simulink model "model_2020b"  (R2020b)
settings: Solver=VariableStepAuto  StartTime=0.0  StopTime=time  MaxStep=1e-3  RelTol=1e-3
values from neighbouring files (symbols this model uses):
  adj_mtx = zeros(N,N)    [main.m]
  c = 1/denominator    [main.m]
  K = B' * P / R    [main.m]
  leader_controller = place(A,B,poles)    [main.m]
  png_vector = [1 0 0 0 0 0]    [main.m]
  selected_signal = 2    [main.m]
libraries: cstblocks x8, simulink x1
settings Model: Creator=salvo  LastModifiedBy=salvo
settings DebuggingCC: UnconnectedInputMsg=none  UnconnectedOutputMsg=none  UnconnectedLineMsg=none  SFMachineParentedDataDiag=error

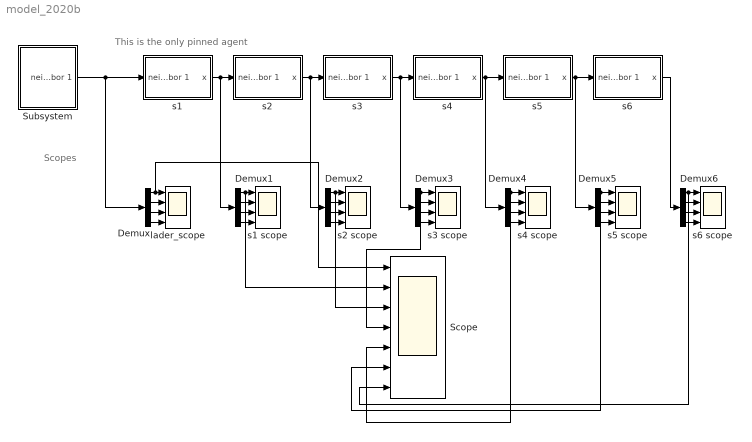
== system model_2020b ==
  note: Scopes
  note: This is the only pinned agent
  Demux{,1..6} (7 alike) : Demux
  Scope : Scope  NumInputPorts=7
  Subsystem : Subsystem
  lader_scope : Scope  NumInputPorts=4
  s1 : Subsystem
  s1 scope : Scope  NumInputPorts=4
  s2 : Subsystem
  s2 scope : Scope  NumInputPorts=4
  s3 : Subsystem
  s3 scope : Scope  NumInputPorts=4
  s4 : Subsystem
  s4 scope : Scope  NumInputPorts=4
  s5 : Subsystem
  s5 scope : Scope  NumInputPorts=4
  s6 : Subsystem
  s6 scope : Scope  NumInputPorts=4
  wires:
  Demux/1 -> Scope/1, lader_scope/1
  Demux/2 -> lader_scope/2
  Demux/3 -> lader_scope/3
  Demux/4 -> lader_scope/4
  Demux1/1 -> Scope/2, s1 scope/1
  Demux1/3 -> s1 scope/3
  Demux1/4 -> s1 scope/4
  Demux1/2 -> s1 scope/2
  s1/1(x) -> Demux1/1, s2/1(neighbor 1)
  Demux2/3 -> s2 scope/3
  Demux2/2 -> s2 scope/2
  s2/1(x) -> Demux2/1, s3/1(neighbor 1)
  Demux2/1 -> Scope/3, s2 scope/1
  Demux2/4 -> s2 scope/4
  Demux3/3 -> s3 scope/3
  Demux3/2 -> s3 scope/2
  s3/1(x) -> Demux3/1, s4/1(neighbor 1)
  Demux3/1 -> Scope/4, s3 scope/1
  Demux3/4 -> s3 scope/4
  Demux4/1 -> Scope/5, s4 scope/1
  Demux4/3 -> s4 scope/3
  s4/1(x) -> Demux4/1, s5/1(neighbor 1)
  Demux4/2 -> s4 scope/2
  Demux4/4 -> s4 scope/4
  Demux5/3 -> s5 scope/3
  s5/1(x) -> Demux5/1, s6/1(neighbor 1)
  Demux5/4 -> s5 scope/4
  Demux5/2 -> s5 scope/2
  Demux5/1 -> Scope/6, s5 scope/1
  Demux6/3 -> s6 scope/3
  Demux6/1 -> Scope/7, s6 scope/1
  s6/1(x) -> Demux6/1
  Demux6/4 -> s6 scope/4
  Demux6/2 -> s6 scope/2
  Subsystem/1(neighbor 1) -> s1/1(neighbor 1), Demux/1

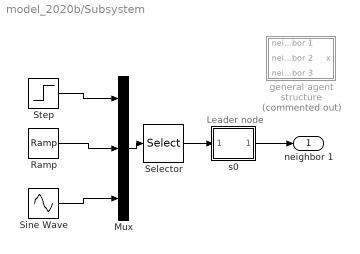
== system model_2020b/Subsystem ==
  note: Leader node
  Mux : Mux  Inputs=3
  Ramp : simulink/Sources/Ramp  slope=1  start=0  InitialOutput=0
  Selector : Selector  InputPortWidth=3  IndexOptions=Index vector (dialog)  Indices=[selected_signal]  OutputSizes=1
  Sine Wave : Sin  Amplitude=10  SampleTime=0
  Step : Step  After=2.5  SampleTime=0
  general agent structure : Subsystem  Commented=on
  s0 : Subsystem
  neighbor 1 : Outport
  wires:
  Sine Wave/1 -> Mux/3
  Selector/1 -> s0/1(In1)
  Step/1 -> Mux/1
  Mux/1 -> Selector/1
  s0/1(neighbor 1) -> neighbor 1/1
  Ramp/1 -> Mux/2

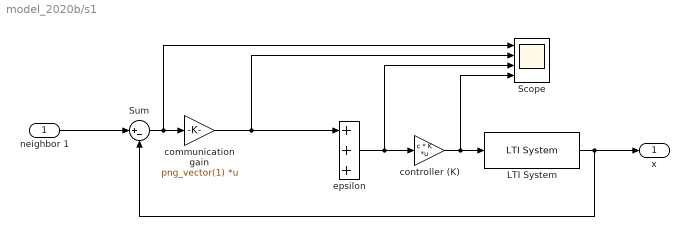
== system model_2020b/s1 ==
  neighbor 1 : Inport
  LTI System : cstblocks/LTI System  sys=sys  IC=x0_1
  Scope : Scope  NumInputPorts=4
  Sum : Sum  Inputs=|+-
  communication gain : Gain  Gain=png_vector(1)  Multiplication=Matrix(K*u)
  controller (K) : Gain  Gain=c * K  Multiplication=Matrix(K*u)
  epsilon : Sum  Inputs=+++
  x : Outport
  wires:
  LTI System/1 -> Sum/2, x/1
  controller (K)/1 -> Scope/4, LTI System/1
  neighbor 1/1 -> Sum/1
  Sum/1 -> Scope/1, communication gain/1
  epsilon/1 -> Scope/3, controller (K)/1
  communication gain/1 -> Scope/2, epsilon/1

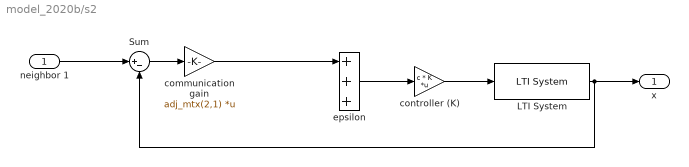
== system model_2020b/s2 ==
  neighbor 1 : Inport
  LTI System : cstblocks/LTI System  sys=sys  IC=x0_2
  Sum : Sum  Inputs=|+-
  communication gain : Gain  Gain=adj_mtx(2,1)  Multiplication=Matrix(K*u)
  controller (K) : Gain  Gain=c * K  Multiplication=Matrix(K*u)
  epsilon : Sum  Inputs=+++
  x : Outport
  wires:
  LTI System/1 -> Sum/2, x/1
  controller (K)/1 -> LTI System/1
  neighbor 1/1 -> Sum/1
  Sum/1 -> communication gain/1
  epsilon/1 -> controller (K)/1
  communication gain/1 -> epsilon/1

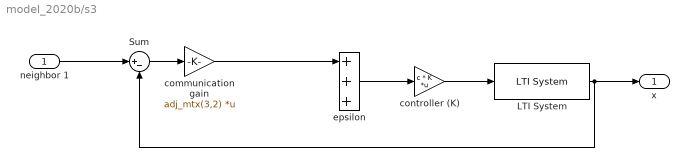
== system model_2020b/s3 ==
  neighbor 1 : Inport
  LTI System : cstblocks/LTI System  sys=sys  IC=x0_3
  Sum : Sum  Inputs=|+-
  communication gain : Gain  Gain=adj_mtx(3,2)  Multiplication=Matrix(K*u)
  controller (K) : Gain  Gain=c * K  Multiplication=Matrix(K*u)
  epsilon : Sum  Inputs=+++
  x : Outport
  wires:
  LTI System/1 -> Sum/2, x/1
  controller (K)/1 -> LTI System/1
  neighbor 1/1 -> Sum/1
  Sum/1 -> communication gain/1
  epsilon/1 -> controller (K)/1
  communication gain/1 -> epsilon/1

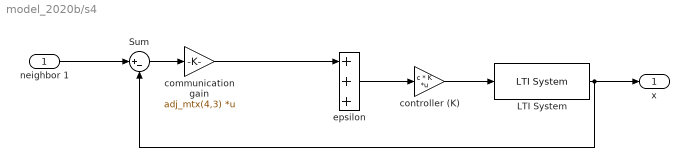
== system model_2020b/s4 ==
  neighbor 1 : Inport
  LTI System : cstblocks/LTI System  sys=sys  IC=x0_4
  Sum : Sum  Inputs=|+-
  communication gain : Gain  Gain=adj_mtx(4,3)  Multiplication=Matrix(K*u)
  controller (K) : Gain  Gain=c * K  Multiplication=Matrix(K*u)
  epsilon : Sum  Inputs=+++
  x : Outport
  wires:
  LTI System/1 -> Sum/2, x/1
  controller (K)/1 -> LTI System/1
  neighbor 1/1 -> Sum/1
  Sum/1 -> communication gain/1
  epsilon/1 -> controller (K)/1
  communication gain/1 -> epsilon/1

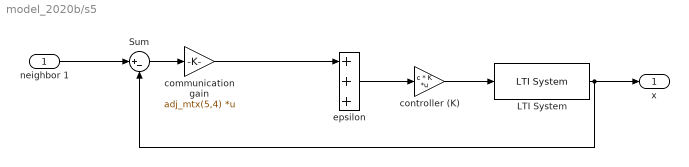
== system model_2020b/s5 ==
  neighbor 1 : Inport
  LTI System : cstblocks/LTI System  sys=sys  IC=x0_5
  Sum : Sum  Inputs=|+-
  communication gain : Gain  Gain=adj_mtx(5,4)  Multiplication=Matrix(K*u)
  controller (K) : Gain  Gain=c * K  Multiplication=Matrix(K*u)
  epsilon : Sum  Inputs=+++
  x : Outport
  wires:
  LTI System/1 -> Sum/2, x/1
  controller (K)/1 -> LTI System/1
  neighbor 1/1 -> Sum/1
  Sum/1 -> communication gain/1
  epsilon/1 -> controller (K)/1
  communication gain/1 -> epsilon/1

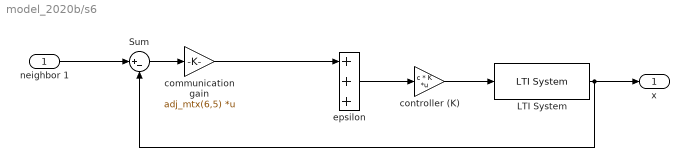
== system model_2020b/s6 ==
  neighbor 1 : Inport
  LTI System : cstblocks/LTI System  sys=sys  IC=x0_6
  Sum : Sum  Inputs=|+-
  communication gain : Gain  Gain=adj_mtx(6,5)  Multiplication=Matrix(K*u)
  controller (K) : Gain  Gain=c * K  Multiplication=Matrix(K*u)
  epsilon : Sum  Inputs=+++
  x : Outport
  wires:
  LTI System/1 -> Sum/2, x/1
  controller (K)/1 -> LTI System/1
  neighbor 1/1 -> Sum/1
  Sum/1 -> communication gain/1
  epsilon/1 -> controller (K)/1
  communication gain/1 -> epsilon/1

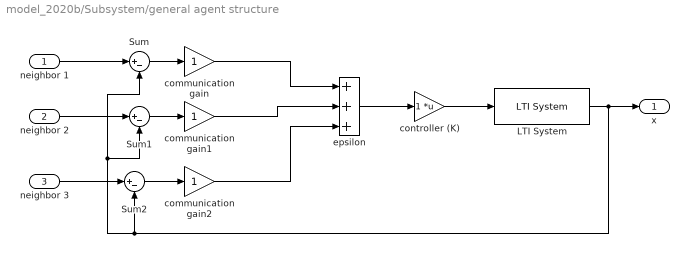
== system model_2020b/Subsystem/general agent structure ==
  neighbor 1 : Inport
  neighbor 2 : Inport  Port=2
  neighbor 3 : Inport  Port=3
  LTI System : cstblocks/LTI System  sys=sys  IC=[]
  Sum : Sum  Inputs=|+-
  Sum1 : Sum  Inputs=|+-
  Sum2 : Sum  Inputs=|+-
  communication gain : Gain
  communication gain1 : Gain
  communication gain2 : Gain
  controller (K) : Gain  Multiplication=Matrix(K*u)
  epsilon : Sum  Inputs=+++
  x : Outport
  wires:
  LTI System/1 -> Sum1/2, Sum/2, Sum2/2, x/1
  controller (K)/1 -> LTI System/1
  neighbor 1/1 -> Sum/1
  Sum/1 -> communication gain/1
  epsilon/1 -> controller (K)/1
  Sum1/1 -> communication gain1/1
  neighbor 2/1 -> Sum1/1
  neighbor 3/1 -> Sum2/1
  Sum2/1 -> communication gain2/1
  communication gain/1 -> epsilon/1
  communication gain1/1 -> epsilon/2
  communication gain2/1 -> epsilon/3

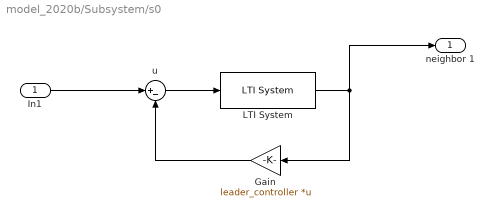
== system model_2020b/Subsystem/s0 ==
  In1 : Inport
  Gain : Gain  Gain=leader_controller  Multiplication=Matrix(K*u)
  LTI System : cstblocks/LTI System  sys=leader_sys  IC=leader_x0
  u : Sum  Inputs=|+-
  neighbor 1 : Outport
  wires:
  LTI System/1 -> neighbor 1/1, Gain/1
  In1/1 -> u/1
  Gain/1 -> u/2
  u/1 -> LTI System/1
